simulink model "A02_L8"  (R2014b)
settings: Solver=ode45  StartTime=0.0  StopTime=10.0  RelTol=1e-3
values from neighbouring files (symbols this model uses):
  h = 0.126    [A03_L8_script.m]
libraries: simulink x1
settings Model: Creator=User  LastModifiedBy=User

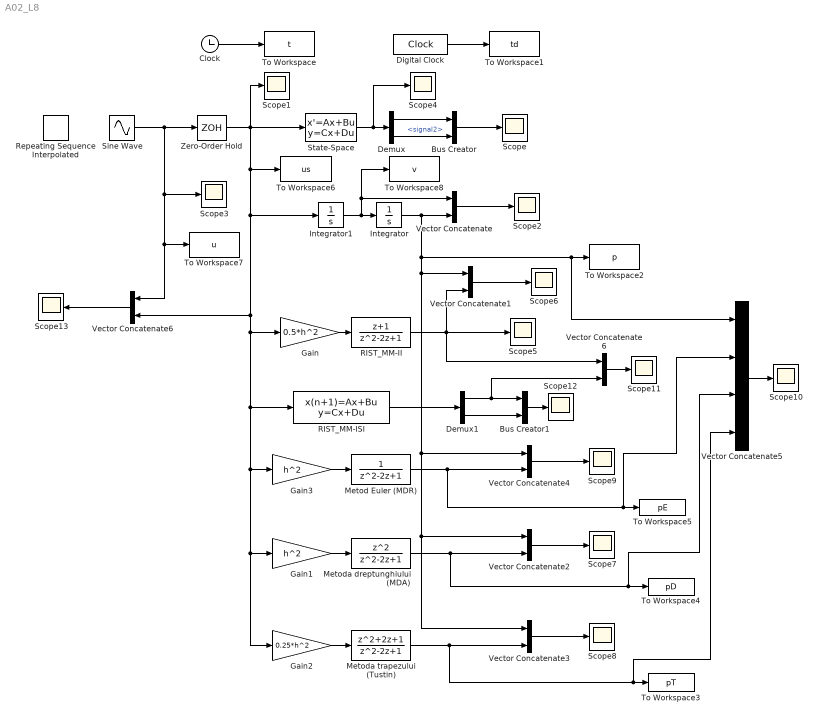
== system A02_L8 ==
  Bus Creator : BusCreator  Inputs=2
  Bus Creator1 : BusCreator  Inputs=2
  Clock : Clock
  Demux : Demux  Outputs=2
  Demux1 : Demux  Outputs=2
  Digital Clock : DigitalClock  SampleTime=h
  Gain : Gain  Gain=0.5*h^2
  Gain1 : Gain  Gain=h^2
  Gain2 : Gain  Gain=0.25*h^2
  Gain3 : Gain  Gain=h^2
  Integrator : Integrator
  Integrator1 : Integrator
  Metod Euler (MDR) : DiscreteTransferFcn  Denominator=[1 -2 1]  SampleTime=h
  Metoda dreptunghiului (MDA) : DiscreteTransferFcn  Numerator=[1 0 0]  Denominator=[1 -2 1]  SampleTime=h
  Metoda trapezului (Tustin) : DiscreteTransferFcn  Numerator=[1 2 1]  Denominator=[1 -2 1]  SampleTime=h
  RIST_MM-II : DiscreteTransferFcn  Numerator=[1 1]  Denominator=[1 -2 1]  SampleTime=h
  RIST_MM-ISI : DiscreteStateSpace  A=[1 h; 0 1]  B=[0.5*h^2; h]  C=[1 0; 0 1]  D=[0; 0]  X0=[0 ; 0]  SampleTime=h
  Repeating Sequence Interpolated : simulink/Sources/Repeating Sequence Interpolated  OutValues=[3 1 4 2 1].'  TimeValues=[0 0.1 0.5 0.6 1].'  LookUpMeth=Interpolation-Use End Values  tsamp=0.01  OutMin=[]  OutMax=[]  OutDataTypeStr=double  OutputDataTypeScalingMode=double  OutDataType=fixdt(0,8)  OutScaling=2^-10
  Scope{,1..13} (14 alike) : Scope
      Scope10 settings: TickLabels=on  ShowLegends=on  TimeRange=10  YMin=0  YMax=120  SaveName=ScopeData10  MaxDataPoints=50000  SampleInput=on
      Scope11 settings: SaveName=ScopeData11  MaxDataPoints=50000
      Scope12 settings: SaveName=ScopeData12
      Scope13 settings: TickLabels=on  ShowLegends=on  TimeRange=10  YMin=0.8  YMax=4.2  SaveName=intrari  MaxDataPoints=50000
      Scope2 settings: SaveName=ScopeData2
      Scope3 settings: SaveName=ScopeData3
      Scope4 settings: SaveName=ScopeData4
      Scope5 settings: SaveName=ScopeData5
      Scope6 settings: ShowLegends=on  SaveName=ScopeData6  MaxDataPoints=50000
      Scope7 settings: SaveName=ScopeData7  MaxDataPoints=50000
      Scope8 settings: SaveName=ScopeData8  MaxDataPoints=50000
      Scope9 settings: SaveName=ScopeData9  MaxDataPoints=50000
  Sine Wave : Sin  Amplitude=5  Frequency=4*pi  Phase=0.1  SampleTime=0
  State-Space : StateSpace  A=[0 1;0 0]  B=[0; 1]  C=[1 0;0 1]  D=[0;0]  X0=[0; 0]
  To Workspace : ToWorkspace  VariableName=t  SampleTime=-1
  To Workspace1 : ToWorkspace  VariableName=td  SampleTime=h
  To Workspace2 : ToWorkspace  VariableName=p  SampleTime=h
  To Workspace3 : ToWorkspace  VariableName=pT  SampleTime=h
  To Workspace4 : ToWorkspace  VariableName=pD  SampleTime=h
  To Workspace5 : ToWorkspace  VariableName=pE  SampleTime=h
  To Workspace6 : ToWorkspace  VariableName=us  SaveFormat=Timeseries  SampleTime=h
  To Workspace7 : ToWorkspace  VariableName=u  SaveFormat=Timeseries  SampleTime=-1
  To Workspace8 : ToWorkspace  VariableName=v  SampleTime=-1
  Vector Concatenate{,1..4,6} (6 alike) : Concatenate
  Vector Concatenate 6 : Concatenate
  Vector Concatenate5 : Concatenate  NumInputs=4
  Zero-Order Hold : ZeroOrderHold  SampleTime=h
  wires:
  Zero-Order Hold/1 -> State-Space/1, Scope1/1, To Workspace6/1, Gain2/1, Gain1/1, Gain3/1, RIST_MM-ISI/1, Gain/1, Vector Concatenate6/2, Integrator1/1
  Integrator1/1 -> To Workspace8/1, Vector Concatenate/1, Integrator/1
  Clock/1 -> To Workspace/1
  Digital Clock/1 -> To Workspace1/1
  Vector Concatenate/1 -> Scope2/1
  Bus Creator/1 -> Scope/1
  State-Space/1 -> Demux/1, Scope4/1
  Demux/2 -> Bus Creator/2  "<signal2>"
  Demux/1 -> Bus Creator/1
  Gain/1 -> RIST_MM-II/1
  Vector Concatenate1/1 -> Scope6/1
  Gain1/1 -> Metoda dreptunghiului (MDA)/1
  Integrator/1 -> Vector Concatenate4/1, Vector Concatenate2/1, Vector Concatenate3/1, Vector Concatenate1/1, Vector Concatenate5/1, To Workspace2/1, Vector Concatenate/2
  Vector Concatenate2/1 -> Scope7/1
  Gain2/1 -> Metoda trapezului (Tustin)/1
  Metoda trapezului (Tustin)/1 -> Vector Concatenate5/4, To Workspace3/1, Vector Concatenate3/2
  Vector Concatenate3/1 -> Scope8/1
  Gain3/1 -> Metod Euler (MDR)/1
  Vector Concatenate4/1 -> Scope9/1
  Vector Concatenate5/1 -> Scope10/1
  Metoda dreptunghiului (MDA)/1 -> Vector Concatenate5/3, To Workspace4/1, Vector Concatenate2/2
  Metod Euler (MDR)/1 -> Vector Concatenate5/2, To Workspace5/1, Vector Concatenate4/2
  RIST_MM-II/1 -> Vector Concatenate 6/1, Scope5/1, Vector Concatenate1/2
  Vector Concatenate 6/1 -> Scope11/1
  Demux1/2 -> Bus Creator1/2
  RIST_MM-ISI/1 -> Demux1/1
  Demux1/1 -> Vector Concatenate 6/2, Bus Creator1/1
  Bus Creator1/1 -> Scope12/1
  Vector Concatenate6/1 -> Scope13/1
  Sine Wave/1 -> Scope3/1, To Workspace7/1, Vector Concatenate6/1, Zero-Order Hold/1
